simulink model "clv1d"  (Simulink 3.00)
settings: Solver=ode45  SolverMode=SingleTasking  StartTime=0.0  StopTime=40  RelTol=1e-3  AbsTol=1e-6
settings Model: ExternalInput=[]  SaveTime=off  SaveOutput=off  InitialState=[]  IntegerOverflowMsg=none  RTWOptions="-aEnforceIntegerDowncast=1 -aFoldNonRolledExpr=1 -aInlineInvariantSignals=1 -aInlineParameters=0 -aLocalBlockOutputs=1 -aRollThreshold=5 -aZeroInternalMemoryAtStartup=1 -aZeroExternalMemoryAtStartup=1 -aInitFltsAndDblsToZero=1 -aGenerateReport=0 -aGenCodeOnly=0 -aRTWVerbose=1 -aIncludeHyperlinkInReport=0 -aLaunchReport=0 -aForceParamTrailComments=0 -aGenerateComments=1 -aIgnoreCustomStorageClasses=1 -aIncHierarchyInIds=0 -aMaxRTWIdLen=31 -aShowEliminatedStatements=0 -aPrefixModelToSubsysFcnNames=1 -aIncDataTypeInIds=0 -aInsertBlockDesc=0 -aSimulinkBlockComments=1 -aInlinedPrmAccess=\"Literals\"  -aSuppressErrorStatus=0 -aModelReferenceCompliant=1 -aSupportNonInlinedSFcns=1 -aSupportContinuousTime=1 -aSupportComplex=1 -aSupportNonFinite=1 -aSupportAbsoluteTime=1 -aTargetFcnLib=\"ansi_tfl_tmw.mat\" -aMultiInstanceERTCode=0 -aLogVarNameModifier=\"rt_\" -aIsPILTarget=0 -aCombineOutputUpdateFcns=0 -aGenerateASAP2=0 -aGenerateSampleERTMain=0 -aGenerateFullHeader=1 -aUtilityFuncGeneration=\"Auto\" -aIncludeFileDelimiter=\"Auto\" -aIncludeMdlTerminateFcn=1 -aPurelyIntegerCode=0 -aERTCustomFileBanners=0 -aRTWCAPIStates=0 -aRTWCAPIParams=0 -aRTWCAPISignals=0 -aMatFileLogging=1 -aGenFloatMathFcnCalls=\"ANSI_C\" -aExtModeMexFile=\"ext_comm\" -aExtModeTransport=0 -aExtModeStaticAllocSize=1000000 -aExtModeTesting=0 -aExtModeStaticAlloc=0 -aExtMode=0  -aInitFltsAndDblsToZero=1 -aInitFltsAndDblsToZero=1 -aInitFltsAndDblsToZero=1"  Creator=The MathWorks Inc.  LastModifiedBy=gcampa

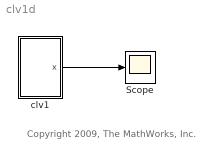
== system clv1d ==
  note: Copyright 2009, The MathWorks, Inc.
  Scope : Scope
      settings: TimeRange=40  YMin=0  YMax=6  SaveToWorkspace=off  SaveName=ScopeData
  clv1 : Subsystem  mask(Competitive Lotka Volterra System){A=0.2, R=0.5, x0=0.1}
      mask prompts: x0 "Initial Condition"
      mask help:
      | This autonomous system represents the competitive lotka volterra system
      |  xdot =  Rx .* ( 1 - Ax)
      |  where each component of x represents a population,
      |  A is an interaction matrix, and R is a diagonal "growth rate" matrix.
      |  Parameters and initial state can be selected from the mask.
      mask Help:
      | This autonomous system represents the competitive lotka volterra system
      |  <p>
      |  The system equations are:
      |  xdot =  Rx .* ( 1 - Ax)
      |  where each component of x represents a population,
      |  A is an interaction matrix, and R is a diagonal "growth rate" matrix.
      |  Parameters and initial state can be selected from the mask.
  wires:
  clv1/1(x) -> Scope/1

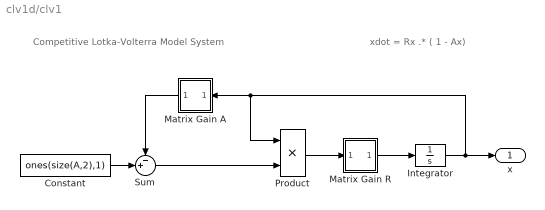
== system clv1d/clv1 ==
  note: Competitive Lotka-Volterra Model System
  note: xdot = Rx .* ( 1 - Ax)
  Constant : Constant  Value=ones(size(A,2),1)
  Integrator : Integrator  ExternalReset=none  InitialConditionSource=internal  InitialCondition=x0  LimitOutput=off  UpperSaturationLimit=inf  LowerSaturationLimit=-inf  ShowSaturationPort=off  ShowStatePort=off  AbsoluteTolerance=auto
  Matrix Gain A : Subsystem  Orientation=left  mask(Matrix Gain){K=A}
      mask prompts: K "Gain matrix:"
      mask help: Matrix Gain.
      mask Help: Multiplies input vector by entered matrix to produce output vector (y=Au).
      mask Display: disp('A')
  Matrix Gain R : Subsystem  mask(Matrix Gain){K=R}
      mask prompts: K "Gain matrix:"
      mask help: Matrix Gain.
      mask Help: Multiplies input vector by entered matrix to produce output vector (y=Au).
      mask Display: disp('R')
  Product : Product  Inputs=2  SaturateOnIntegerOverflow=on
  Sum : Sum  Inputs=-+|  SaturateOnIntegerOverflow=off
  x : Outport  Port=1
  wires:
  Constant/1 -> Sum/2
  Matrix Gain A/1(Out1) -> Sum/1
  Sum/1 -> Product/2
  Integrator/1 -> x/1, Product/1, Matrix Gain A/1(In1)
  Product/1 -> Matrix Gain R/1(In1)
  Matrix Gain R/1(Out1) -> Integrator/1

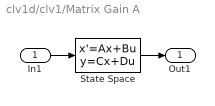
== system clv1d/clv1/Matrix Gain A ==
  In1 : Inport  Port=1  PortWidth=-1  SampleTime=-1  DataType=auto
      settings: SignalType=auto
  State Space : StateSpace  A=[]  B=[]  C=[]  D=K  X0=0
  Out1 : Outport  Port=1
  wires:
  In1/1 -> State Space/1
  State Space/1 -> Out1/1

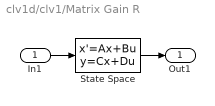
== system clv1d/clv1/Matrix Gain R ==
  In1 : Inport  Port=1  PortWidth=-1  SampleTime=-1  DataType=auto
      settings: SignalType=auto
  State Space : StateSpace  A=[]  B=[]  C=[]  D=K  X0=0
  Out1 : Outport  Port=1
  wires:
  State Space/1 -> Out1/1
  In1/1 -> State Space/1
